simulink model "Copy_of_dinamica_estabilidad2017b"  (R2017b)
settings: Solver=ode45  StartTime=0.0  StopTime=100  RelTol=1e-3
values from neighbouring files (symbols this model uses):
  k = dlqr(A_barra,B_barra,Q,R)    [LQR.m]
  r = 7.5e-2    (= 0.075)    [LQR.m]
  Ts = 1/200    (= 0.005)    [LQR.m]
libraries: cstblocks x2
settings Model: Creator=raulD
settings SolverCC: ZeroCrossAlgorithm=Adaptive
settings DataIOCC: ReturnWorkspaceOutputs=on
settings DebuggingCC: UnconnectedInputMsg=none  UnconnectedOutputMsg=none  UnconnectedLineMsg=none
settings ModelReferenceCC: EnableRefExpFcnMdlSchedulingChecks=off
settings SFSimCC: SimUseLocalCustomCode=on
settings RTWCC: Description=Generic Real-Time Target  RTWUseLocalCustomCode=on

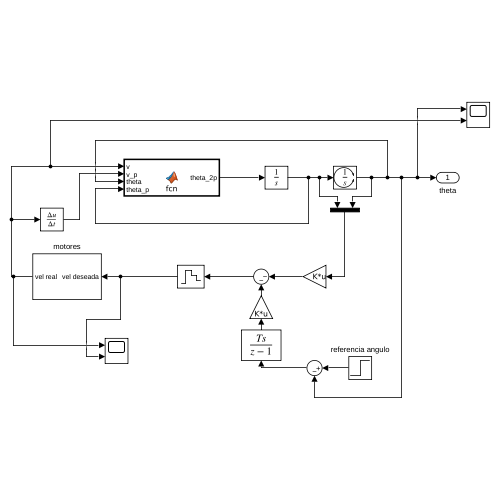
[thumbnail: Simulink's stored preview of the top-level diagram]
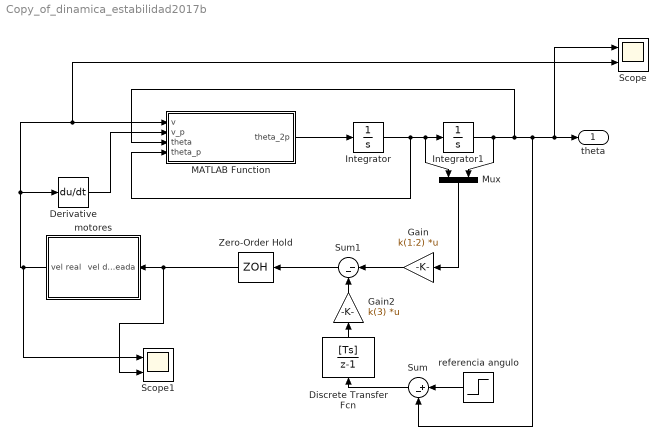
== system Copy_of_dinamica_estabilidad2017b ==
  Derivative : Derivative
  Discrete Transfer Fcn : DiscreteTransferFcn  Numerator=[Ts]  Denominator=[1 -1]  SampleTime=Ts
  Gain : Gain  Gain=k(1:2)  Multiplication=Matrix(K*u)
  Gain2 : Gain  Gain=k(3)  Multiplication=Matrix(K*u)
  Integrator : Integrator  InitialCondition=0.1  ContinuousStateAttributes='w'
  Integrator1 : Integrator  InitialCondition=1*pi/180  WrapState=on  WrappedStateUpperValue=pi/2  WrappedStateLowerValue=-pi/2  ContinuousStateAttributes='theta'
  MATLAB Function : MATLAB Function  TreatAsAtomicUnit=on
  Mux : Mux  Inputs=2
  Scope : Scope  NumInputPorts=2
  Scope1 : Scope  NumInputPorts=2
  Sum : Sum  Inputs=|+-
  Sum1 : Sum  Inputs=|--
  Zero-Order Hold : ZeroOrderHold  SampleTime=Ts
  motores : Subsystem
  referencia angulo : Step  Time=10  After=0.5*pi/180  SampleTime=0
  theta : Outport
  wires:
  MATLAB Function/1(theta_2p) -> Integrator/1
  Integrator/1 -> Mux/1, Integrator1/1, MATLAB Function/4(theta_p)
  Derivative/1 -> MATLAB Function/2(v_p)
  Mux/1 -> Gain/1
  motores/1(vel real) -> Scope1/1, Scope/2, MATLAB Function/1(v), Derivative/1
  Integrator1/1 -> Mux/2, MATLAB Function/3(theta), Sum/2, Scope/1, theta/1
  referencia angulo/1 -> Sum/1
  Sum/1 -> Discrete Transfer Fcn/1
  Discrete Transfer Fcn/1 -> Gain2/1
  Gain2/1 -> Sum1/2
  Gain/1 -> Sum1/1
  Zero-Order Hold/1 -> Scope1/2, motores/1(vel deseada)
  Sum1/1 -> Zero-Order Hold/1

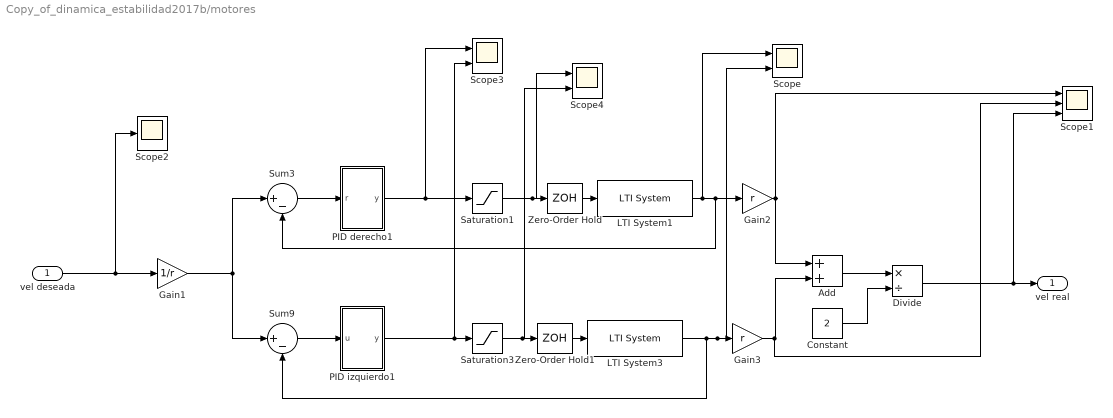
== system Copy_of_dinamica_estabilidad2017b/motores ==
  vel deseada : Inport
  Add : Sum
  Constant : Constant  Value=2
  Divide : Product  Inputs=*/
  Gain1 : Gain  Gain=1/r
  Gain2 : Gain  Gain=r
  Gain3 : Gain  Gain=r
  LTI System1 : cstblocks/LTI System  sys=tf_vel_drch  IC=[]
  LTI System3 : cstblocks/LTI System  sys=tf_vel_izq  IC=[]
  PID derecho1 : Subsystem
  PID izquierdo1 : Subsystem
  Saturation1 : Saturate  UpperLimit=100  LowerLimit=-100
  Saturation3 : Saturate  UpperLimit=100  LowerLimit=-100
  Scope : Scope  NumInputPorts=2
  Scope1 : Scope  NumInputPorts=3
  Scope2 : Scope
  Scope3 : Scope  NumInputPorts=2
  Scope4 : Scope  NumInputPorts=2
  Sum3 : Sum  Inputs=|+-
  Sum9 : Sum  Inputs=|+-
  Zero-Order Hold : ZeroOrderHold  SampleTime=1/500
  Zero-Order Hold1 : ZeroOrderHold  SampleTime=1/500
  vel real : Outport
  wires:
  LTI System1/1 -> Scope/1, Gain2/1, Sum3/2
  Sum9/1 -> PID izquierdo1/1(u)
  PID derecho1/1(y) -> Scope3/1, Saturation1/1
  LTI System3/1 -> Scope/2, Gain3/1, Sum9/2
  Saturation1/1 -> Scope4/1, Zero-Order Hold/1
  Gain1/1 -> Sum9/1, Sum3/1
  Sum3/1 -> PID derecho1/1(r)
  Constant/1 -> Divide/2
  PID izquierdo1/1(y) -> Scope3/2, Saturation3/1
  Saturation3/1 -> Scope4/2, Zero-Order Hold1/1
  Add/1 -> Divide/1
  Gain3/1 -> Add/2, Scope1/2
  vel deseada/1 -> Scope2/1, Gain1/1
  Gain2/1 -> Scope1/1, Add/1
  Divide/1 -> Scope1/3, vel real/1
  Zero-Order Hold/1 -> LTI System1/1
  Zero-Order Hold1/1 -> LTI System3/1

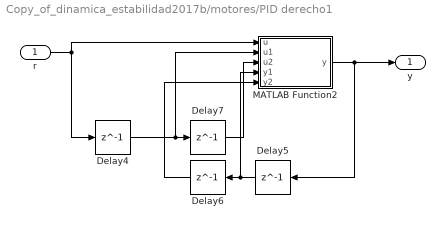
== system Copy_of_dinamica_estabilidad2017b/motores/PID derecho1 ==
  r : Inport
  Delay{4..7} (4 alike) : Delay  DelayLength=1  InitialCondition=0  SampleTime=1/500
  MATLAB Function2 : MATLAB Function  TreatAsAtomicUnit=on
  y : Outport
  wires:
  Delay5/1 -> MATLAB Function2/4(y1), Delay6/1
  Delay4/1 -> MATLAB Function2/2(u1), Delay7/1
  Delay7/1 -> MATLAB Function2/3(u2)
  Delay6/1 -> MATLAB Function2/5(y2)
  r/1 -> Delay4/1, MATLAB Function2/1(u)
  MATLAB Function2/1(y) -> y/1, Delay5/1

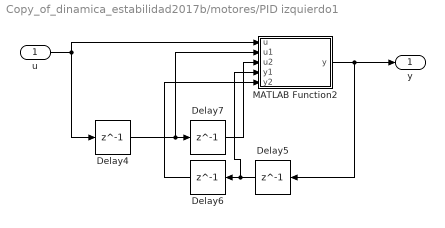
== system Copy_of_dinamica_estabilidad2017b/motores/PID izquierdo1 ==
  u : Inport
  Delay{4..7} (4 alike) : Delay  DelayLength=1  InitialCondition=0  SampleTime=1/500
  MATLAB Function2 : MATLAB Function  TreatAsAtomicUnit=on
  y : Outport
  wires:
  MATLAB Function2/1(y) -> Delay5/1, y/1
  u/1 -> MATLAB Function2/1(u), Delay4/1
  Delay6/1 -> MATLAB Function2/5(y2)
  Delay7/1 -> MATLAB Function2/3(u2)
  Delay4/1 -> Delay7/1, MATLAB Function2/2(u1)
  Delay5/1 -> Delay6/1, MATLAB Function2/4(y1)

== matlab function Copy_of_dinamica_estabilidad2017b/MATLAB Function ==
  data: theta_2p output; v input; v_p input; theta input; theta_p input
function theta_2p = fcn(v, v_p, theta, theta_p)

g = 9.8;
L = 20e-2;
beta_v = 0.2;
M = 40e-2;
m = 1;

theta_2p = (g*m*sin(theta) - m*v_p*cos(theta) - 2*beta_v*v*cos(theta) + m*v_p*cos(theta)^3 + m*cos(theta)^2*sin(theta) - M*v_p*cos(theta) + M*g*sin(theta) + 2*L*m*theta_p^2*cos(theta)*sin(theta))/(L*(- m*cos(theta)^2 + M + m));

== matlab function Copy_of_dinamica_estabilidad2017b/motores/PID derecho1/MATLAB Function2 ==
  data: u input; y output; u1 input; u2 input; y1 input; y2 input
function y = fcn(u, u1, u2, y1, y2)

y = 13.72619*u-26.86414*u1+13.14425*u2+1.96944*y1-0.96944*y2;

== matlab function Copy_of_dinamica_estabilidad2017b/motores/PID izquierdo1/MATLAB Function2 ==
  data: u input; y output; u1 input; u2 input; y1 input; y2 input
function y = fcn(u, u1, u2, y1, y2)

y = 9.0799*u-17.72430*u1+8.64954*u2+1.96425*y1-0.96425*y2;
